simulink model "TST_SfFunctionWithBusTypes"  (Simulink 10.0)
settings: Solver=FixedStepDiscrete  StartTime=0.0  StopTime=10.0  FixedStep=0.02  RelTol=1e-3  EnableMultiTasking=on
settings Model: Creator=kharthforeign  LastModifiedBy=unknown
settings DataIOCC: LimitDataPoints=on  SignalLoggingSaveFormat=ModelDataLogs  SaveOutput=off  SignalLogging=off  SaveTime=off
settings OptimizationCC: BlockReduction=off  ConditionallyExecuteInputs=off  OptimizeBlockIOStorage=off  BufferReuse=off  GlobalBufferReuse=off  ExpressionFolding=off  ExpressionDepthLimit=2147483647  LocalBlockOutputs=off  InitFltsAndDblsToZero=on  OptimizeDataStoreBuffers=off  BusAssignmentInplaceUpdate=off
settings DebuggingCC: SolverPrmCheckMsg=warning  FcnCallInpInsideContextMsg=warning  StateNameClashWarn=warning
settings SFSimCC: SimParseCustomCode=off
settings GRTTargetCC: GeneratePreprocessorConditionals=Disable all
settings ConfigComp: CovExternalEMLEnable=off

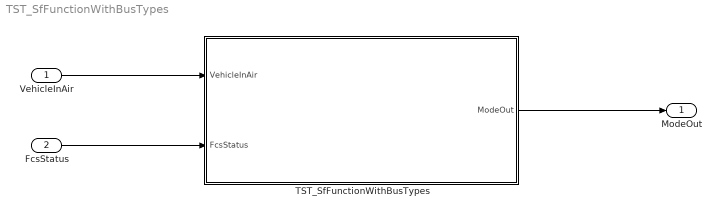
== system TST_SfFunctionWithBusTypes ==
  VehicleInAir : Inport  OutDataTypeStr=boolean  PortDimensions=1
  FcsStatus : Inport  Port=2  OutDataTypeStr=Bus: FCS_FlightControlSystem_Status
  TST_SfFunctionWithBusTypes : Subsystem  TreatAsAtomicUnit=on
  ModeOut : Outport  OutDataTypeStr=uint32  PortDimensions=1
  wires:
  VehicleInAir/1 -> TST_SfFunctionWithBusTypes/1(VehicleInAir)
  FcsStatus/1 -> TST_SfFunctionWithBusTypes/2(FcsStatus)
  TST_SfFunctionWithBusTypes/1(ModeOut) -> ModeOut/1

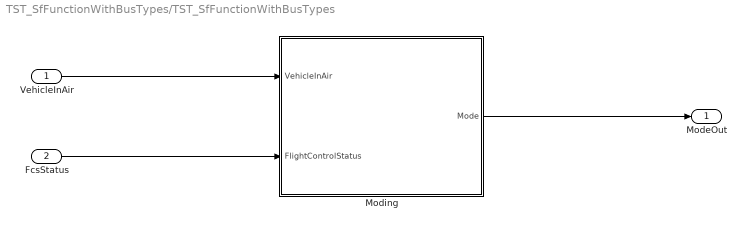
== system TST_SfFunctionWithBusTypes/TST_SfFunctionWithBusTypes ==
  VehicleInAir : Inport  OutDataTypeStr=boolean  PortDimensions=1
  FcsStatus : Inport  Port=2  OutDataTypeStr=Bus: FCS_FlightControlSystem_Status
  Moding : Stateflow chart  TreatAsAtomicUnit=on
  ModeOut : Outport  OutDataTypeStr=uint32  PortDimensions=1
  wires:
  FcsStatus/1 -> Moding/2(FlightControlStatus)
  VehicleInAir/1 -> Moding/1(VehicleInAir)
  Moding/1(Mode) -> ModeOut/1

== stateflow chart TST_SfFunctionWithBusTypes/Moding ==
  state UpdateFeedthroughParameters(FcsStatusInput) [function]
    (default) -> (junction 6)
    (junction 6) -> (junction 7) [order 1] : [FcsStatusInput.PressureAltitude_Ft > 5000.0]...
        | {Mode = uint32(5);}
    (junction 6) -> (junction 8) [order 2] : {Mode = uint32(5);}
  state Main
    entry:
    UpdateFeedthroughParameters(FlightControlStatus);
  (default) -> Main
  data: FcsStatusInput function_input FCS_FlightControlSystem_Status; VehicleInAir input boolean; Mode output uint32; FlightControlStatus input FCS_FlightControlSystem_Status
